simulink library "libMdl_quatToEuler"  (R2019b)
settings: Solver=VariableStepAuto  StartTime=0.0  StopTime=10.0  RelTol=1e-3
settings Model: Creator=hwinter  LastModifiedBy=Hanno
settings DataIOCC: ReturnWorkspaceOutputs=off
settings DebuggingCC: ArithmeticOperatorsInVariantConditions=warning
settings SFSimCC: SimUseLocalCustomCode=off  CustomCodeUndefinedFunction=UseInterfaceOnly
settings RTWCC: RTWUseLocalCustomCode=off

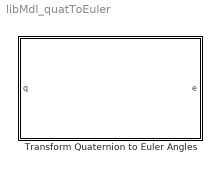
== system libMdl_quatToEuler ==
  Transform Quaternion to Euler Angles : Subsystem
      mask Display:
      | color('black')
      | text(0.5,0.5,'Rotation order: ZYX','horizontalAlignment', 'center')

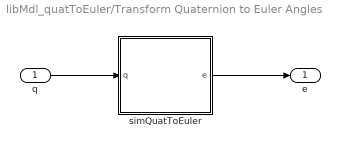
== system libMdl_quatToEuler/Transform Quaternion to Euler Angles ==
  q : Inport
  simQuatToEuler : MATLAB Function  TreatAsAtomicUnit=on
  e : Outport  VectorParamsAs1DForOutWhenUnconnected=off
  wires:
  simQuatToEuler/1(e) -> e/1
  q/1 -> simQuatToEuler/1(q)

== matlab function libMdl_quatToEuler/Transform Quaternion to Euler Angles/simQuatToEuler ==
  data: q input; e output
function e = simQuatToEuler(q)

e = quatToEuler(q);

end % function
